simulink model "cop"  (R2020a)
settings: Solver=FixedStepAuto  StartTime=0.0  StopTime=300  FixedStep=1  RelTol=1e-3
undefined symbols (not defined in the file or in its folder): inf_depth, Kc_ini, PGravel
libraries: simulink x4
(part 2 of 2)

== system cop/COP/Climate Model/ Final Calculation for Data/Wind Speed/Wind Speed measured at 2m height (u2) [m//s] ==
  uz : Inport
  z : Inport  Port=2
  Constant : Constant  Value=4.87
  Constant1 : Constant  Value=67.8
  Constant2 : Constant  Value=5.42
  Divide : Product  Inputs=**/
  Math Function : Math  Operator=log  SaturateOnIntegerOverflow=on
  Product : Product
  Subtract : Sum  Inputs=+-
  u2 : Outport
  wires:
  uz/1 -> Divide/1
  Constant/1 -> Divide/2
  Math Function/1 -> Divide/3
  z/1 -> Product/2
  Constant1/1 -> Product/1
  Product/1 -> Subtract/1
  Subtract/1 -> Math Function/1
  Constant2/1 -> Subtract/2
  Divide/1 -> u2/1

== system cop/COP/Soil Model/Dual Crop Coefficient (Kcb + Ke)/Crop Basal Component/Adjustment to Crop Coefficient ==
  Constant2 : Constant  Value=0.3
  Constant3 : Constant  Value=3
  Constant4 : Constant  Value=0.004
  Constant5 : Constant  Value=45
  Constant6 : Constant  Value=0.04
  Constant7 : Constant  Value=2
  Divide : Product  Inputs=*/
  Math Function : Math  Operator=pow  SaturateOnIntegerOverflow=on
  Product : Product
  Product1 : Product
  Product2 : Product
  Subtract : Sum  Inputs=+-
  Subtract1 : Sum  Inputs=+-
  Subtract2 : Sum  Inputs=+-
  Kcb_adj : Outport
  wires:
  Product/1 -> Kcb_adj/1
  Subtract/1 -> Product/1
  [u2] -> Subtract2/1
  Constant4/1 -> Product1/1
  Constant7/1 -> Subtract2/2
  [RHmin] -> Subtract1/1
  Product1/1 -> Subtract/2
  Constant5/1 -> Subtract1/2
  Divide/1 -> Math Function/1
  Constant3/1 -> Divide/2
  Constant2/1 -> Math Function/2
  Product2/1 -> Subtract/1
  [MaxCropHatStage] -> Divide/1
  Subtract2/1 -> Product2/2
  Math Function/1 -> Product/2
  Subtract1/1 -> Product1/2
  Constant6/1 -> Product2/1

== system cop/COP/Soil Model/Dual Crop Coefficient (Kcb + Ke)/Crop Basal Component/Development Stage ==
  Kcb ini : Inport
  Kcb mid : Inport  Port=2
  Add : Sum
  Divide : Product  Inputs=*/
  Product : Product
  Subtract : Sum  Inputs=+-
  Subtract1 : Sum  Inputs=+-
  Out1 : Outport
  wires:
  Add/1 -> Out1/1
  Kcb ini/1 -> Add/1, Subtract/2
  Product/1 -> Add/2
  Subtract/1 -> Product/2
  Kcb mid/1 -> Subtract/1
  Divide/1 -> Product/1
  [Ldev] -> Divide/2
  Subtract1/1 -> Divide/1
  [Lini] -> Subtract1/2
  [DafterPD] -> Subtract1/1

== system cop/COP/Soil Model/Dual Crop Coefficient (Kcb + Ke)/Crop Basal Component/Late Season Stage ==
  Kcb mid : Inport
  Kcb_adj : Inport  Port=2
  Add : Sum
  Add1 : Sum
  Add2 : Sum  Inputs=+++
  Divide : Product  Inputs=*/
  Product : Product
  Subtract : Sum  Inputs=+-
  Subtract1 : Sum  Inputs=+-
  Out1 : Outport
  wires:
  [Kcb_end] -> Add/1
  Kcb_adj/1 -> Add/2
  Subtract/1 -> Product/2
  Divide/1 -> Product/1
  [DafterPD] -> Subtract1/1
  Add1/1 -> Out1/1
  Product/1 -> Add1/2
  [Llate] -> Divide/2
  Kcb mid/1 -> Add1/1, Subtract/2
  Subtract1/1 -> Divide/1
  Add/1 -> Subtract/1
  Add2/1 -> Subtract1/2
  [Lini] -> Add2/1
  [Ldev] -> Add2/2
  [Lmid] -> Add2/3

== system cop/COP/Soil Model/Dual Crop Coefficient (Kcb + Ke)/Crop Basal Component/Mid-season Stage ==
  Kcb_adj : Inport
  Add : Sum
  Constant : Constant  Value=0
  Switch : Switch  Criteria=u2 > Threshold  Threshold=0.45
  Kcb mid : Outport
  wires:
  Add/1 -> Kcb mid/1
  [Kcb_mid] -> Add/1, Switch/2
  Kcb_adj/1 -> Switch/1
  Switch/1 -> Add/2
  Constant/1 -> Switch/3

== system cop/COP/Soil Model/Dual Crop Coefficient (Kcb + Ke)/Evaporation Component/Exposed and wetted soil fraction (few) ==
  Constant1 : Constant
  Effective fraction of soil surface covered by vegetation fc : Subsystem
  Min : MinMax  Inputs=2
  Subtract : Sum  Inputs=+-
  Out1 : Outport
  wires:
  Min/1 -> Out1/1
  Subtract/1 -> Min/1
  [fw] -> Min/2
  Constant1/1 -> Subtract/1
  Effective fraction of soil surface covered by vegetation fc/1(Out1) -> Subtract/2

== system cop/COP/Soil Model/Dual Crop Coefficient (Kcb + Ke)/Evaporation Component/Soil evaporation reduction coefficient (Kr) ==
  De_i Daily Water Balance [mm] : Subsystem
  Delay : Delay  DelayLength=1  InitialConditionSource=Input port  InitialCondition=0
      settings: InputPortMap=u0,p4
  Display : Display
  Divide : Product  Inputs=*/
  REWmax total readily evaporable water [mm] : Subsystem
  Subtract : Sum  Inputs=+-
  Subtract1 : Sum  Inputs=+-
  TEWmax total evaporable water [mm] : Subsystem
  initial De_i-1 value : Constant  Value=0
  Out1 : Outport
  tag scope: De_past=global, REW=global, TEW=global
  wires:
  Divide/1 -> Out1/1
  TEWmax total evaporable water [mm]/1(Out1) -> Display/1, [TEW], Subtract/1, Subtract1/1
  Subtract/1 -> Divide/1
  Subtract1/1 -> Divide/2
  REWmax total readily evaporable water [mm]/1(Out1) -> [REW], Subtract1/2
  [De_past] -> Subtract/2
  De_i Daily Water Balance [mm]/1(Out1) -> Delay/1
  Delay/1 -> De_i Daily Water Balance [mm]/1(De_past), [De_past]
  initial De_i-1 value/1 -> Delay/2

== system cop/COP/Soil Model/Dual Crop Coefficient (Kcb + Ke)/Evaporation Component/Upper Limit (Kc max) ==
  Kcb : Inport
  0.05 : Constant  Value=0.05
  Add : Sum
  Add1 : Sum
  Adjustment to Crop Coefficient : Subsystem
  Constant : Constant  Value=1.2
  MinMax : MinMax  Function=max  Inputs=2
  Out1 : Outport
  wires:
  MinMax/1 -> Out1/1
  Constant/1 -> Add/1
  Adjustment to Crop Coefficient/1(Kcb_adj) -> Add/2
  Add/1 -> MinMax/1
  Kcb/1 -> Add1/1
  Add1/1 -> MinMax/2
  0.05/1 -> Add1/2

== system cop/COP/Soil Model/Reference Evapotraspiration (ET0) [mm//day]/Actual Vapor Pressure (ea) [kPa]/Derived from Dewpoint Temperature ==
  Saturation Vapor Pressure (eo) : Subsystem
  Out1 : Outport
  wires:
  [Tdew] -> Saturation Vapor Pressure (eo)/1(In1)
  Saturation Vapor Pressure (eo)/1(Out1) -> Out1/1

== system cop/COP/Soil Model/Reference Evapotraspiration (ET0) [mm//day]/Actual Vapor Pressure (ea) [kPa]/Derived from Psychrometric Data ==
  Constant : Constant  Value=apsy
  Product : Product
  Product1 : Product
  Saturation Vapor Pressure (eo) : Subsystem
  Subtract : Sum  Inputs=+-
  Subtract1 : Sum  Inputs=+-
  Out1 : Outport
  wires:
  Subtract/1 -> Out1/1
  Saturation Vapor Pressure (eo)/1(Out1) -> Subtract/1
  [Twet] -> Subtract1/2, Saturation Vapor Pressure (eo)/1(In1)
  [Tdry] -> Subtract1/1
  Subtract1/1 -> Product/1
  Product/1 -> Subtract/2
  Product1/1 -> Product/2
  [AP] -> Product1/2
  Constant/1 -> Product1/1

== system cop/COP/Soil Model/Reference Evapotraspiration (ET0) [mm//day]/Actual Vapor Pressure (ea) [kPa]/Derived from RHmax & RHmin ==
  Add : Sum
  Constant : Constant  Value=100
  Constant1 : Constant  Value=2
  Constant2 : Constant  Value=100
  Divide : Product  Inputs=**/
  Divide1 : Product  Inputs=**/
  Divide2 : Product  Inputs=*/
  Saturation Vapor Pressure (eo) : Subsystem
  Saturation Vapor Pressure (eo)1 : Subsystem
  Out1 : Outport
  wires:
  Divide2/1 -> Out1/1
  [Tmin] -> Saturation Vapor Pressure (eo)/1(In1)
  Saturation Vapor Pressure (eo)/1(Out1) -> Divide/1
  [RHmax] -> Divide/2
  Constant/1 -> Divide/3
  Divide/1 -> Add/1
  Divide1/1 -> Add/2
  Add/1 -> Divide2/1
  Constant1/1 -> Divide2/2
  Constant2/1 -> Divide1/3
  [RHmin] -> Divide1/2
  [Tmax] -> Saturation Vapor Pressure (eo)1/1(In1)
  Saturation Vapor Pressure (eo)1/1(Out1) -> Divide1/1

== system cop/COP/Soil Model/Reference Evapotraspiration (ET0) [mm//day]/Actual Vapor Pressure (ea) [kPa]/Derived from RHmax only ==
  Constant : Constant  Value=100
  Divide : Product  Inputs=**/
  Saturation Vapor Pressure (eo) : Subsystem
  Out1 : Outport
  wires:
  Constant/1 -> Divide/3
  [Tmin] -> Saturation Vapor Pressure (eo)/1(In1)
  [RHmax] -> Divide/2
  Saturation Vapor Pressure (eo)/1(Out1) -> Divide/1
  Divide/1 -> Out1/1

== system cop/COP/Soil Model/Reference Evapotraspiration (ET0) [mm//day]/Actual Vapor Pressure (ea) [kPa]/Derived from RHmean only ==
  Add : Sum
  Constant : Constant  Value=2
  Constant1 : Constant  Value=100
  Divide : Product  Inputs=*/
  Divide1 : Product  Inputs=*/
  Product : Product
  Saturation Vapor Pressure (eo) : Subsystem
  Saturation Vapor Pressure (eo)1 : Subsystem
  Out1 : Outport
  wires:
  [Tmax] -> Saturation Vapor Pressure (eo)/1(In1)
  Saturation Vapor Pressure (eo)/1(Out1) -> Add/1
  Saturation Vapor Pressure (eo)1/1(Out1) -> Add/2
  [Tmin] -> Saturation Vapor Pressure (eo)1/1(In1)
  Add/1 -> Divide/1
  Constant/1 -> Divide/2
  Divide/1 -> Product/2
  [RHmean] -> Divide1/1
  Constant1/1 -> Divide1/2
  Divide1/1 -> Product/1
  Product/1 -> Out1/1

== system cop/COP/Soil Model/Reference Evapotraspiration (ET0) [mm//day]/Mean Saturation Vapor Pressure (es) [kPa] /Saturation Vapor Pressure (eo) ==
  In1 : Inport
  Add : Sum
  Constant : Constant  Value=0.6108
  Constant1 : Constant  Value=17.27
  Constant2 : Constant  Value=237.3
  Divide : Product  Inputs=**/
  Math Function : Math  SaturateOnIntegerOverflow=on
  Product : Product
  Out1 : Outport
  wires:
  Product/1 -> Out1/1
  Constant1/1 -> Divide/1
  In1/1 -> Add/1, Divide/2
  Add/1 -> Divide/3
  Divide/1 -> Math Function/1
  Constant/1 -> Product/1
  Constant2/1 -> Add/2
  Math Function/1 -> Product/2

== system cop/COP/Soil Model/Reference Evapotraspiration (ET0) [mm//day]/Mean Saturation Vapor Pressure (es) [kPa] /Saturation Vapor Pressure (eo) 2 ==
  In1 : Inport
  Add1 : Sum
  Constant3 : Constant  Value=0.6108
  Constant4 : Constant  Value=17.27
  Constant5 : Constant  Value=237.3
  Divide1 : Product  Inputs=**/
  Math Function1 : Math  SaturateOnIntegerOverflow=on
  Product1 : Product
  Out1 : Outport
  wires:
  Math Function1/1 -> Product1/2
  Constant4/1 -> Divide1/1
  Add1/1 -> Divide1/3
  Constant3/1 -> Product1/1
  Divide1/1 -> Math Function1/1
  In1/1 -> Divide1/2, Add1/1
  Product1/1 -> Out1/1
  Constant5/1 -> Add1/2

== system cop/COP/Soil Model/Reference Evapotraspiration (ET0) [mm//day]/Psychrometric Constant (Y) [kPA//°C]/Latent Heat of Vaporization (l) [MJ//kg] ==
  "Latent Heat for an Air Temperature of about 20°C " : Constant  Value=2.45
  l : Outport
  wires:
  "Latent Heat for an Air Temperature of about 20°C "/1 -> l/1

== system cop/COP/Soil Model/Reference Evapotraspiration (ET0) [mm//day]/Soil Heat Flux Density (G) [MJ//m^2//day]/Long Time Steps ==
  Divide : Product  Inputs=**/*
  Subtract : Sum  Inputs=+-
  Out1 : Outport
  wires:
  [cs] -> Divide/1
  [Tmean] -> Subtract/1
  [Tpast] -> Subtract/2
  Subtract/1 -> Divide/2
  [Tpast_t] -> Divide/3
  [Zr] -> Divide/4
  Divide/1 -> Out1/1

== system cop/COP/Soil Model/Soil Data Calculation/Estimated Soil Heat Capacity (UC Davis)/Bulk Density (Saxton and Rawls Function) [g//cm^3) ==
  Add : Sum
  Constant : Constant
  Constant1 : Constant  Value=2.65
  Normal Density (g/cm^3) : Subsystem
  Product : Product
  Product1 : Product
  Subtract : Sum  Inputs=+-
  Volum Fraction of Gravel (g/cm^3) : Subsystem
  Out1 : Outport
  wires:
  Add/1 -> Out1/1
  Normal Density (g/cm^3)/1(Out1) -> Product/1, Volum Fraction of Gravel (g/cm^3)/1(In1)
  Subtract/1 -> Product/2
  Product/1 -> Add/1
  Constant/1 -> Subtract/1
  Product1/1 -> Add/2
  Constant1/1 -> Product1/2
  Volum Fraction of Gravel (g/cm^3)/1(Out1) -> Subtract/2, Product1/1

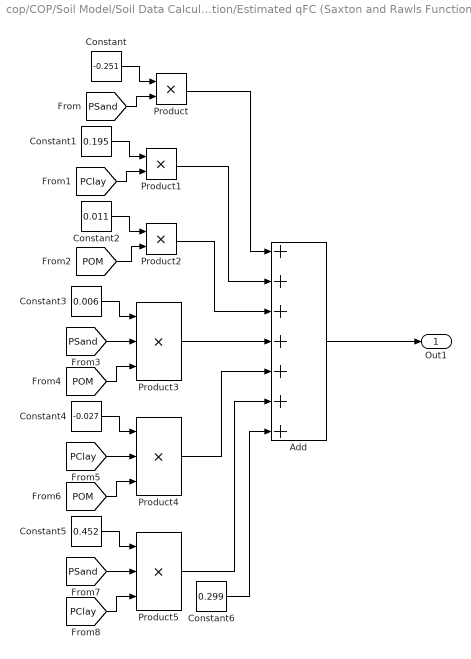
== system cop/COP/Soil Model/Soil Data Calculation/Estimated qFC (Saxton and Rawls Function)/θ33t ==
  Add : Sum  Inputs=+++++++
  Constant : Constant  Value=-0.251
  Constant1 : Constant  Value=0.195
  Constant2 : Constant  Value=0.011
  Constant3 : Constant  Value=0.006
  Constant4 : Constant  Value=-0.027
  Constant5 : Constant  Value=0.452
  Constant6 : Constant  Value=0.299
  Product : Product
  Product1 : Product
  Product2 : Product
  Product3 : Product  Inputs=3
  Product4 : Product  Inputs=3
  Product5 : Product  Inputs=3
  Out1 : Outport
  wires:
  [PClay] -> Product5/3
  [PClay] -> Product1/2
  Constant4/1 -> Product4/1
  Product1/1 -> Add/2
  Constant3/1 -> Product3/1
  Product5/1 -> Add/6
  [PClay] -> Product4/2
  Product4/1 -> Add/5
  Constant6/1 -> Add/7
  Constant5/1 -> Product5/1
  [PSand] -> Product5/2
  Product/1 -> Add/1
  [PSand] -> Product/2
  Product2/1 -> Add/3
  Constant2/1 -> Product2/1
  Constant1/1 -> Product1/1
  Product3/1 -> Add/4
  Constant/1 -> Product/1
  [POM] -> Product2/2
  [PSand] -> Product3/2
  [POM] -> Product4/3
  [POM] -> Product3/3
  Add/1 -> Out1/1

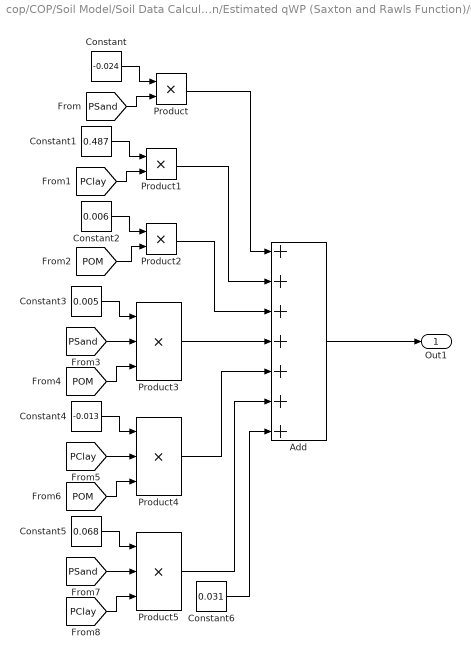
== system cop/COP/Soil Model/Soil Data Calculation/Estimated qWP (Saxton and Rawls Function)/θ1500t ==
  Add : Sum  Inputs=+++++++
  Constant : Constant  Value=-0.024
  Constant1 : Constant  Value=0.487
  Constant2 : Constant  Value=0.006
  Constant3 : Constant  Value=0.005
  Constant4 : Constant  Value=-0.013
  Constant5 : Constant  Value=0.068
  Constant6 : Constant  Value=0.031
  Product : Product
  Product1 : Product
  Product2 : Product
  Product3 : Product  Inputs=3
  Product4 : Product  Inputs=3
  Product5 : Product  Inputs=3
  Out1 : Outport
  wires:
  [PClay] -> Product5/3
  [PClay] -> Product1/2
  Constant4/1 -> Product4/1
  Product1/1 -> Add/2
  Constant3/1 -> Product3/1
  Product5/1 -> Add/6
  [PClay] -> Product4/2
  Product4/1 -> Add/5
  Constant6/1 -> Add/7
  Constant5/1 -> Product5/1
  [PSand] -> Product5/2
  Product/1 -> Add/1
  [PSand] -> Product/2
  Product2/1 -> Add/3
  Constant2/1 -> Product2/1
  Constant1/1 -> Product1/1
  Product3/1 -> Add/4
  Constant/1 -> Product/1
  [POM] -> Product2/2
  [PSand] -> Product3/2
  [POM] -> Product4/3
  [POM] -> Product3/3
  Add/1 -> Out1/1

== system cop/COP/Climate Model/ Final Calculation for Data/Net Radiation at the Crop Surface (Rn) [MJ//m^2//day]/Extraterrestrial Radiation (Ra) [MJ//m^2//day]/Inverse Relative Distance Earth-Sun (dr) ==
  J : Inport
  Add : Sum
  Constant : Constant
  Constant1 : Constant  Value=0.033
  Constant2 : Constant  Value=2*pi
  Divide : Product  Inputs=**/
  Product : Product
  Trigonometric Function : Trigonometry  Operator=cos
  dr : Outport
  wires:
  Add/1 -> dr/1
  Constant/1 -> Add/1
  Product/1 -> Add/2
  Constant1/1 -> Product/1
  Trigonometric Function/1 -> Product/2
  Divide/1 -> Trigonometric Function/1
  Constant2/1 -> Divide/1
  [DinYear] -> Divide/3
  J/1 -> Divide/2

== system cop/COP/Climate Model/ Final Calculation for Data/Net Radiation at the Crop Surface (Rn) [MJ//m^2//day]/Extraterrestrial Radiation (Ra) [MJ//m^2//day]/Latitude in Radian (φ) [rad] ==
  Add : Sum
  Constant : Constant  Value=pi/180
  Constant1 : Constant  Value=60
  Divide : Product  Inputs=*/
  Product : Product
  φ : Outport
  wires:
  Constant/1 -> Product/1
  Add/1 -> Product/2
  [LatDeg] -> Add/1
  [LatMin] -> Divide/1
  Constant1/1 -> Divide/2
  Divide/1 -> Add/2
  Product/1 -> φ/1

== system cop/COP/Climate Model/ Final Calculation for Data/Net Radiation at the Crop Surface (Rn) [MJ//m^2//day]/Extraterrestrial Radiation (Ra) [MJ//m^2//day]/Solar Declination in Radian (δ) [rad] ==
  J : Inport
  Constant1 : Constant  Value=0.409
  Constant2 : Constant  Value=2*pi
  Constant4 : Constant  Value=1.39
  Divide : Product  Inputs=**/
  Product : Product
  Subtract : Sum  Inputs=+-
  Trigonometric Function : Trigonometry
  δ : Outport
  wires:
  [DinYear] -> Divide/3
  Product/1 -> δ/1
  Trigonometric Function/1 -> Product/2
  J/1 -> Divide/2
  Constant2/1 -> Divide/1
  Constant1/1 -> Product/1
  Divide/1 -> Subtract/1
  Subtract/1 -> Trigonometric Function/1
  Constant4/1 -> Subtract/2

== system cop/COP/Climate Model/ Final Calculation for Data/Net Radiation at the Crop Surface (Rn) [MJ//m^2//day]/Extraterrestrial Radiation (Ra) [MJ//m^2//day]/Sunset Hour Angle (Ws) [rad] ==
  Constant : Constant  Value=-1
  Product : Product  Inputs=3
  Trigonometric Function : Trigonometry  Operator=acos
  Trigonometric Function1 : Trigonometry  Operator=tan
  Trigonometric Function2 : Trigonometry  Operator=tan
  Ws : Outport
  wires:
  Trigonometric Function/1 -> Ws/1
  Product/1 -> Trigonometric Function/1
  Constant/1 -> Product/1
  Trigonometric Function1/1 -> Product/2
  Trigonometric Function2/1 -> Product/3
  [LatRad] -> Trigonometric Function1/1
  [SolDec] -> Trigonometric Function2/1

== system cop/COP/Climate Model/ Final Calculation for Data/Net Radiation at the Crop Surface (Rn) [MJ//m^2//day]/Net Solar//Shortwave Radiation (Rns) [MJ//m^2//day]/Albedo or canopy reflection coefficient for the reference crop (G) ==
  Constant : Constant  Value=0.23
  Out1 : Outport
  wires:
  Constant/1 -> Out1/1

== system cop/COP/Climate Model/ Final Calculation for Data/Net Radiation at the Crop Surface (Rn) [MJ//m^2//day]/Solar Radiation (Rs) [MJ//m^2//day]/Angstrom Formula if AI_Rs not avaliable ==
  In1 : Inport
  Add : Sum
  Default as : Constant  Value=0.25
  Default bs : Constant  Value=0.50
  Divide : Product  Inputs=**/
  Maximum Daylight Hour (N) [hour] : Subsystem
  Product : Product
  Out1 : Outport
  wires:
  Default as/1 -> Add/1
  Default bs/1 -> Divide/1
  Divide/1 -> Add/2
  In1/1 -> Divide/2
  Add/1 -> Product/1
  Product/1 -> Out1/1
  [Ra] -> Product/2
  Maximum Daylight Hour (N) [hour]/1(N) -> Divide/3

== system cop/COP/Climate Model/ Final Calculation for Data/Net Radiation at the Crop Surface (Rn) [MJ//m^2//day]/Solar Radiation (Rs) [MJ//m^2//day]/Hargreaves Formula if AI_Rs and hour of daylight is not available ==
  Constant : Constant  Value=kRs
  Product : Product  Inputs=3
  Sqrt : Sqrt  SaturateOnIntegerOverflow=on
  Subtract : Sum  Inputs=+-
  Rs : Outport
  wires:
  Product/1 -> Rs/1
  Constant/1 -> Product/1
  [Ra] -> Product/3
  Sqrt/1 -> Product/2
  Subtract/1 -> Sqrt/1
  [Tmin] -> Subtract/2
  [Tmax] -> Subtract/1

== system cop/COP/Soil Model/Dual Crop Coefficient (Kcb + Ke)/Evaporation Component/Exposed and wetted soil fraction (few)/Effective fraction of soil surface covered by vegetation fc ==
  Constant : Constant
  Constant1 : Constant  Value=0.5
  Constant2 : Constant  Value=0.01
  Divide : Product  Inputs=*/
  Math Function : Math  Operator=pow  SaturateOnIntegerOverflow=on
  MinMax : MinMax  Function=max  Inputs=2
  Product : Product
  Subtract : Sum  Inputs=+-
  Subtract1 : Sum  Inputs=+-
  Subtract2 : Sum
  Out1 : Outport
  wires:
  Divide/1 -> Math Function/1
  [Kcb] -> Subtract/1
  [Kcb_ini] -> Subtract1/2, Subtract/2
  Subtract/1 -> MinMax/2
  [Kc_max] -> Subtract1/1
  Subtract1/1 -> Divide/2
  Subtract2/1 -> Math Function/2
  Constant/1 -> Subtract2/1
  Product/1 -> Subtract2/2
  Constant1/1 -> Product/1
  [Ph] -> Product/2
  Math Function/1 -> Out1/1
  MinMax/1 -> Divide/1
  Constant2/1 -> MinMax/1

== system cop/COP/Soil Model/Dual Crop Coefficient (Kcb + Ke)/Evaporation Component/Soil evaporation reduction coefficient (Kr)/De_i Daily Water Balance [mm] ==
  De_past : Inport
  Constant : Constant  Value=0
  Constant1 : Constant  Value=0
  Deep Percolation DPe [mm/day] : Subsystem
  Divide : Product  Inputs=*/
  Divide1 : Product  Inputs=*/
  MinMax : MinMax  Inputs=2
  MinMax1 : MinMax  Function=max  Inputs=2
  MinMax2 : MinMax  Function=max  Inputs=2
  Subtract : Sum  Inputs=+--+++
  Subtract1 : Sum  Inputs=+-
  Out1 : Outport
  wires:
  De_past/1 -> Subtract/1
  Subtract/1 -> MinMax/1
  [P] -> Subtract1/1
  [RO] -> Subtract1/2
  Subtract1/1 -> Subtract/2
  [I] -> Divide/1
  Divide/1 -> Subtract/3
  [fw] -> Divide/2
  Divide1/1 -> Subtract/4
  [E] -> Divide1/1
  [few] -> Divide1/2
  [Te] -> Subtract/5
  Deep Percolation DPe [mm/day]/1(Out1) -> MinMax2/1
  MinMax/1 -> MinMax1/1
  MinMax1/1 -> Out1/1
  [TEW] -> MinMax/2
  Constant/1 -> MinMax1/2
  Constant1/1 -> MinMax2/2
  MinMax2/1 -> Subtract/6

== system cop/COP/Soil Model/Dual Crop Coefficient (Kcb + Ke)/Evaporation Component/Soil evaporation reduction coefficient (Kr)/REWmax total readily evaporable water [mm] ==
  MABIA Method : Subsystem
  Manual Switch : ManualSwitch  CurrentSetting=0
  Ritchie et al. (1989) : Subsystem
  Out1 : Outport
  wires:
  MABIA Method/1(Out1) -> Manual Switch/2
  Ritchie et al. (1989)/1(Out1) -> Manual Switch/1
  Manual Switch/1 -> Out1/1

== system cop/COP/Soil Model/Dual Crop Coefficient (Kcb + Ke)/Evaporation Component/Soil evaporation reduction coefficient (Kr)/TEWmax total evaporable water [mm] ==
  Constant : Constant  Value=1000
  Constant1 : Constant  Value=0.5
  Product : Product  Inputs=3
  Product1 : Product
  Subtract : Sum  Inputs=+-
  Out1 : Outport
  wires:
  Product/1 -> Out1/1
  Constant/1 -> Product/1
  Subtract/1 -> Product/2
  [qFC] -> Subtract/1
  Product1/1 -> Subtract/2
  [qWP] -> Product1/2
  Constant1/1 -> Product1/1
  [Ze] -> Product/3

== system cop/COP/Soil Model/Dual Crop Coefficient (Kcb + Ke)/Evaporation Component/Upper Limit (Kc max)/Adjustment to Crop Coefficient ==
  Constant2 : Constant  Value=0.3
  Constant3 : Constant  Value=3
  Constant4 : Constant  Value=0.004
  Constant5 : Constant  Value=45
  Constant6 : Constant  Value=0.04
  Constant7 : Constant  Value=2
  Divide : Product  Inputs=*/
  Math Function : Math  Operator=pow  SaturateOnIntegerOverflow=on
  Product : Product
  Product1 : Product
  Product2 : Product
  Subtract : Sum  Inputs=+-
  Subtract1 : Sum  Inputs=+-
  Subtract2 : Sum  Inputs=+-
  Kcb_adj : Outport
  wires:
  Product/1 -> Kcb_adj/1
  Subtract/1 -> Product/1
  [u2] -> Subtract2/1
  Constant4/1 -> Product1/1
  Constant7/1 -> Subtract2/2
  [RHmin] -> Subtract1/1
  Product1/1 -> Subtract/2
  Constant5/1 -> Subtract1/2
  Divide/1 -> Math Function/1
  Constant3/1 -> Divide/2
  Constant2/1 -> Math Function/2
  Product2/1 -> Subtract/1
  [MaxCropHatStage] -> Divide/1
  Subtract2/1 -> Product2/2
  Math Function/1 -> Product/2
  Subtract1/1 -> Product1/2
  Constant6/1 -> Product2/1

== system cop/COP/Soil Model/Reference Evapotraspiration (ET0) [mm//day]/Actual Vapor Pressure (ea) [kPa]/Derived from Dewpoint Temperature/Saturation Vapor Pressure (eo) ==
  In1 : Inport
  Add : Sum
  Constant : Constant  Value=0.6108
  Constant1 : Constant  Value=17.27
  Constant2 : Constant  Value=237.3
  Divide : Product  Inputs=**/
  Math Function : Math  SaturateOnIntegerOverflow=on
  Product : Product
  Out1 : Outport
  wires:
  Product/1 -> Out1/1
  Constant1/1 -> Divide/1
  In1/1 -> Add/1, Divide/2
  Add/1 -> Divide/3
  Divide/1 -> Math Function/1
  Constant/1 -> Product/1
  Constant2/1 -> Add/2
  Math Function/1 -> Product/2

== system cop/COP/Soil Model/Reference Evapotraspiration (ET0) [mm//day]/Actual Vapor Pressure (ea) [kPa]/Derived from Psychrometric Data/Saturation Vapor Pressure (eo) ==
  In1 : Inport
  Add : Sum
  Constant : Constant  Value=0.6108
  Constant1 : Constant  Value=17.27
  Constant2 : Constant  Value=237.3
  Divide : Product  Inputs=**/
  Math Function : Math  SaturateOnIntegerOverflow=on
  Product : Product
  Out1 : Outport
  wires:
  Product/1 -> Out1/1
  Constant1/1 -> Divide/1
  In1/1 -> Add/1, Divide/2
  Add/1 -> Divide/3
  Divide/1 -> Math Function/1
  Constant/1 -> Product/1
  Constant2/1 -> Add/2
  Math Function/1 -> Product/2

== system cop/COP/Soil Model/Reference Evapotraspiration (ET0) [mm//day]/Actual Vapor Pressure (ea) [kPa]/Derived from RHmax & RHmin/Saturation Vapor Pressure (eo) ==
  In1 : Inport
  Add : Sum
  Constant : Constant  Value=0.6108
  Constant1 : Constant  Value=17.27
  Constant2 : Constant  Value=237.3
  Divide : Product  Inputs=**/
  Math Function : Math  SaturateOnIntegerOverflow=on
  Product : Product
  Out1 : Outport
  wires:
  Product/1 -> Out1/1
  Constant1/1 -> Divide/1
  In1/1 -> Add/1, Divide/2
  Add/1 -> Divide/3
  Divide/1 -> Math Function/1
  Constant/1 -> Product/1
  Constant2/1 -> Add/2
  Math Function/1 -> Product/2

== system cop/COP/Soil Model/Reference Evapotraspiration (ET0) [mm//day]/Actual Vapor Pressure (ea) [kPa]/Derived from RHmax & RHmin/Saturation Vapor Pressure (eo)1 ==
  In1 : Inport
  Add : Sum
  Constant : Constant  Value=0.6108
  Constant1 : Constant  Value=17.27
  Constant2 : Constant  Value=237.3
  Divide : Product  Inputs=**/
  Math Function : Math  SaturateOnIntegerOverflow=on
  Product : Product
  Out1 : Outport
  wires:
  Math Function/1 -> Product/2
  Constant2/1 -> Add/2
  Constant/1 -> Product/1
  Divide/1 -> Math Function/1
  Add/1 -> Divide/3
  In1/1 -> Divide/2, Add/1
  Constant1/1 -> Divide/1
  Product/1 -> Out1/1

== system cop/COP/Soil Model/Reference Evapotraspiration (ET0) [mm//day]/Actual Vapor Pressure (ea) [kPa]/Derived from RHmax only/Saturation Vapor Pressure (eo) ==
  In1 : Inport
  Add : Sum
  Constant : Constant  Value=0.6108
  Constant1 : Constant  Value=17.27
  Constant2 : Constant  Value=237.3
  Divide : Product  Inputs=**/
  Math Function : Math  SaturateOnIntegerOverflow=on
  Product : Product
  Out1 : Outport
  wires:
  Product/1 -> Out1/1
  Constant1/1 -> Divide/1
  In1/1 -> Add/1, Divide/2
  Add/1 -> Divide/3
  Divide/1 -> Math Function/1
  Constant/1 -> Product/1
  Constant2/1 -> Add/2
  Math Function/1 -> Product/2

== system cop/COP/Soil Model/Reference Evapotraspiration (ET0) [mm//day]/Actual Vapor Pressure (ea) [kPa]/Derived from RHmean only/Saturation Vapor Pressure (eo) ==
  In1 : Inport
  Add : Sum
  Constant : Constant  Value=0.6108
  Constant1 : Constant  Value=17.27
  Constant2 : Constant  Value=237.3
  Divide : Product  Inputs=**/
  Math Function : Math  SaturateOnIntegerOverflow=on
  Product : Product
  Out1 : Outport
  wires:
  Product/1 -> Out1/1
  Constant1/1 -> Divide/1
  In1/1 -> Add/1, Divide/2
  Add/1 -> Divide/3
  Divide/1 -> Math Function/1
  Constant/1 -> Product/1
  Constant2/1 -> Add/2
  Math Function/1 -> Product/2

== system cop/COP/Soil Model/Reference Evapotraspiration (ET0) [mm//day]/Actual Vapor Pressure (ea) [kPa]/Derived from RHmean only/Saturation Vapor Pressure (eo)1 ==
  In1 : Inport
  Add : Sum
  Constant : Constant  Value=0.6108
  Constant1 : Constant  Value=17.27
  Constant2 : Constant  Value=237.3
  Divide : Product  Inputs=**/
  Math Function : Math  SaturateOnIntegerOverflow=on
  Product : Product
  Out1 : Outport
  wires:
  Math Function/1 -> Product/2
  Constant2/1 -> Add/2
  Constant/1 -> Product/1
  Divide/1 -> Math Function/1
  Add/1 -> Divide/3
  In1/1 -> Divide/2, Add/1
  Constant1/1 -> Divide/1
  Product/1 -> Out1/1

== system cop/COP/Soil Model/Soil Data Calculation/Estimated Soil Heat Capacity (UC Davis)/Bulk Density (Saxton and Rawls Function) [g//cm^3)/Normal Density (g//cm^3) ==
  Constant : Constant  Value=2.65
  Constant1 : Constant
  Product : Product
  Saturated Moisture θS : Subsystem
  Subtract : Sum  Inputs=+-
  Out1 : Outport
  wires:
  Product/1 -> Out1/1
  Constant/1 -> Product/2
  Subtract/1 -> Product/1
  Constant1/1 -> Subtract/1
  Saturated Moisture θS/1(Out1) -> Subtract/2

== system cop/COP/Soil Model/Soil Data Calculation/Estimated Soil Heat Capacity (UC Davis)/Bulk Density (Saxton and Rawls Function) [g//cm^3)/Volum Fraction of Gravel (g//cm^3) ==
  In1 : Inport
  Constant : Constant  Value=2.65
  Constant1 : Constant
  Constant2 : Constant
  Divide : Product  Inputs=*/
  Divide1 : Product  Inputs=*/
  Product : Product
  Product1 : Product
  Subtract : Sum  Inputs=+-
  Subtract1 : Sum  Inputs=+-
  Out1 : Outport
  wires:
  In1/1 -> Divide/1
  [PGravel] -> Product1/1, Product/2
  Constant/1 -> Divide/2
  Divide/1 -> Subtract1/2, Product/1
  Product/1 -> Divide1/1
  Subtract/1 -> Divide1/2
  Constant1/1 -> Subtract/1
  Product1/1 -> Subtract/2
  Subtract1/1 -> Product1/2
  Constant2/1 -> Subtract1/1
  Divide1/1 -> Out1/1

== system cop/COP/Climate Model/ Final Calculation for Data/Net Radiation at the Crop Surface (Rn) [MJ//m^2//day]/Solar Radiation (Rs) [MJ//m^2//day]/Angstrom Formula if AI_Rs not avaliable/Maximum Daylight Hour (N) [hour] ==
  Constant : Constant  Value=24
  Constant1 : Constant  Value=pi
  Divide : Product  Inputs=**/
  N : Outport
  wires:
  Divide/1 -> N/1
  [Ws] -> Divide/2
  Constant/1 -> Divide/1
  Constant1/1 -> Divide/3

== system cop/COP/Soil Model/Dual Crop Coefficient (Kcb + Ke)/Evaporation Component/Soil evaporation reduction coefficient (Kr)/De_i Daily Water Balance [mm]/Deep Percolation DPe [mm//day] ==
  Add : Sum  Inputs=++-
  Divide : Product  Inputs=*/
  Subtract : Sum  Inputs=+-
  Out1 : Outport
  wires:
  Divide/1 -> Add/2
  [P] -> Subtract/1
  [RO] -> Subtract/2
  Subtract/1 -> Add/1
  [I] -> Divide/1
  [fw] -> Divide/2
  [De_past] -> Add/3
  Add/1 -> Out1/1

== system cop/COP/Soil Model/Dual Crop Coefficient (Kcb + Ke)/Evaporation Component/Soil evaporation reduction coefficient (Kr)/REWmax total readily evaporable water [mm]/MABIA Method ==
  Add : Sum
  Constant : Constant  Value=3.121
  Constant1 : Constant  Value=22.896
  Product : Product
  Product1 : Product
  Out1 : Outport
  wires:
  Product1/1 -> Out1/1
  Constant/1 -> Product/1
  [TEW] -> Product/2
  Product/1 -> Add/1
  Constant1/1 -> Add/2
  Add/1 -> Product1/1
  [Ze] -> Product1/2

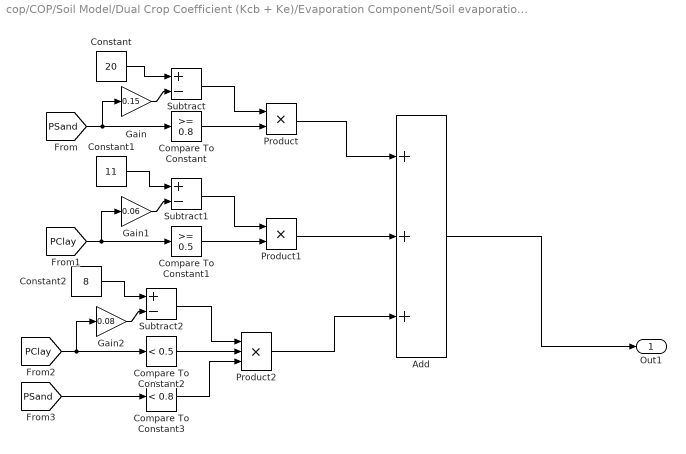
== system cop/COP/Soil Model/Dual Crop Coefficient (Kcb + Ke)/Evaporation Component/Soil evaporation reduction coefficient (Kr)/REWmax total readily evaporable water [mm]/Ritchie et al. (1989) ==
  Add : Sum  Inputs=+++
  Compare To Constant : simulink/Logic and Bit Operations/Compare To Constant  relop=>=  const=0.8  OutDataTypeStr=boolean
  Compare To Constant1 : simulink/Logic and Bit Operations/Compare To Constant  relop=>=  const=0.5  OutDataTypeStr=boolean
  Compare To Constant2 : simulink/Logic and Bit Operations/Compare To Constant  relop=<  const=0.5  OutDataTypeStr=boolean
  Compare To Constant3 : simulink/Logic and Bit Operations/Compare To Constant  relop=<  const=0.8  OutDataTypeStr=boolean
  Constant : Constant  Value=20
  Constant1 : Constant  Value=11
  Constant2 : Constant  Value=8
  Gain : Gain  Gain=0.15
  Gain1 : Gain  Gain=0.06
  Gain2 : Gain  Gain=0.08
  Product : Product
  Product1 : Product
  Product2 : Product  Inputs=3
  Subtract : Sum  Inputs=+-
  Subtract1 : Sum  Inputs=+-
  Subtract2 : Sum  Inputs=+-
  Out1 : Outport
  wires:
  Compare To Constant3/1 -> Product2/3
  [PSand] -> Gain/1, Compare To Constant/1
  Subtract2/1 -> Product2/1
  Product/1 -> Add/1
  Product2/1 -> Add/3
  Gain/1 -> Subtract/2
  Compare To Constant/1 -> Product/2
  Subtract/1 -> Product/1
  Compare To Constant1/1 -> Product1/2
  Constant1/1 -> Subtract1/1
  Subtract1/1 -> Product1/1
  Gain2/1 -> Subtract2/2
  [PClay] -> Compare To Constant1/1, Gain1/1
  Constant2/1 -> Subtract2/1
  [PClay] -> Compare To Constant2/1, Gain2/1
  [PSand] -> Compare To Constant3/1
  Constant/1 -> Subtract/1
  Compare To Constant2/1 -> Product2/2
  Add/1 -> Out1/1
  Product1/1 -> Add/2
  Gain1/1 -> Subtract1/2

== system cop/COP/Soil Model/Soil Data Calculation/Estimated Soil Heat Capacity (UC Davis)/Bulk Density (Saxton and Rawls Function) [g//cm^3)/Normal Density (g//cm^3)/Saturated Moisture θS ==
  Constant : Constant  Value=0.097
  Constant1 : Constant  Value=0.043
  Product : Product
  Subtract : Sum  Inputs=++-+
  θ(S-33) : Subsystem
  Out1 : Outport
  wires:
  Subtract/1 -> Out1/1
  [qFC] -> Subtract/1
  Product/1 -> Subtract/3
  Constant/1 -> Product/1
  [PSand] -> Product/2
  Constant1/1 -> Subtract/4
  θ(S-33)/1(Out1) -> Subtract/2

== system cop/COP/Soil Model/Soil Data Calculation/Estimated Soil Heat Capacity (UC Davis)/Bulk Density (Saxton and Rawls Function) [g//cm^3)/Normal Density (g//cm^3)/Saturated Moisture θS/θ(S-33) ==
  Constant : Constant  Value=0.636
  Constant1 : Constant  Value=0.107
  Product : Product
  Subtract : Sum  Inputs=++-
  θ(S-33)t : Subsystem
  Out1 : Outport
  wires:
  θ(S-33)t/1(Out1) -> Product/1, Subtract/1
  Product/1 -> Subtract/2
  Constant/1 -> Product/2
  Constant1/1 -> Subtract/3
  Subtract/1 -> Out1/1

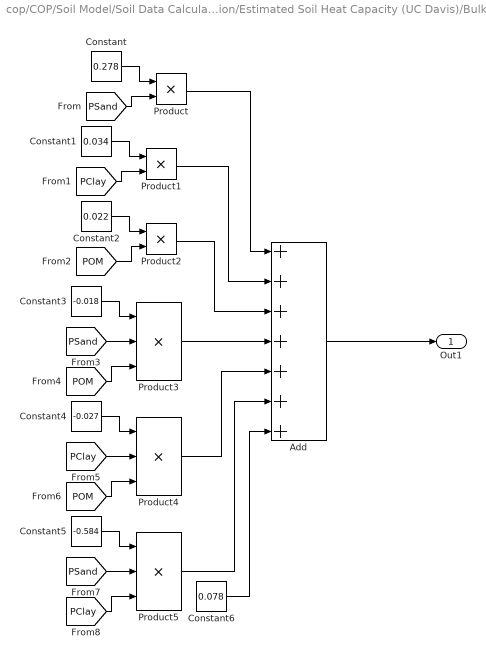
== system cop/COP/Soil Model/Soil Data Calculation/Estimated Soil Heat Capacity (UC Davis)/Bulk Density (Saxton and Rawls Function) [g//cm^3)/Normal Density (g//cm^3)/Saturated Moisture θS/θ(S-33)/θ(S-33)t ==
  Add : Sum  Inputs=+++++++
  Constant : Constant  Value=0.278
  Constant1 : Constant  Value=0.034
  Constant2 : Constant  Value=0.022
  Constant3 : Constant  Value=-0.018
  Constant4 : Constant  Value=-0.027
  Constant5 : Constant  Value=-0.584
  Constant6 : Constant  Value=0.078
  Product : Product
  Product1 : Product
  Product2 : Product
  Product3 : Product  Inputs=3
  Product4 : Product  Inputs=3
  Product5 : Product  Inputs=3
  Out1 : Outport
  wires:
  Add/1 -> Out1/1
  Constant2/1 -> Product2/1
  [POM] -> Product2/2
  Product1/1 -> Add/2
  Product2/1 -> Add/3
  [PClay] -> Product4/2
  Constant3/1 -> Product3/1
  [POM] -> Product3/3
  [PClay] -> Product1/2
  Constant6/1 -> Add/7
  Product5/1 -> Add/6
  [PClay] -> Product5/3
  Product/1 -> Add/1
  Constant5/1 -> Product5/1
  Constant1/1 -> Product1/1
  Constant/1 -> Product/1
  [POM] -> Product4/3
  Product3/1 -> Add/4
  [PSand] -> Product5/2
  [PSand] -> Product3/2
  Constant4/1 -> Product4/1
  [PSand] -> Product/2
  Product4/1 -> Add/5

== matlab function cop/COP/Plant Model/General Plant Database/MATLAB Function1 ==
  data: PDd input; cd output; PDm input; PDy input; DafterPD input; d output; m output; y output
function [cd,d,m,y] = curDate(PDd,PDm,PDy,DafterPD)
    x = datetime(PDy,PDm,PDd);
    x = x + floor(DafterPD);
    xv = datevec(x);
    y = xv(1);
    m = xv(2);
    d = xv(3);
    xm = datetime(y,1,1);
    a = minus(x,xm);
    cd = days(a);
end

== matlab function cop/COP/Plant Model/General Plant Database/MATLAB Function ==
  data: year input; D output
function D = DinYear(year)
    if mod(year, 4) == 0
        D = 366;
        if mod(year, 100) == 0
            D = 365;
            if mod(year,400)==0
                D = 366;
            end
        end
    else
        D = 365;
    end
end

== matlab function cop/COP/Plant Model/Plant Data Calculation/MATLAB Function ==
  data: d input; stage output; Lini input; Ldev input; Lmid input; Llate input
function stage = curPS(d,Lini,Ldev,Lmid,Llate)
    stage = 0;
    d = d - Lini;
    if d <= 0
        return
    end
    stage = 1;
    d = d - Ldev;
    if d <= 0
        return
    end
    stage = 2;
    d = d - Lmid;
    if d <= 0
        return
    end
    stage = 3;
    d = d - Lmid;
    if d <= 0 
        return
    end
    stage = 4;
end

== matlab function cop/COP/Soil Model/General Soil Database/MATLAB Function3 ==
  data: sand input; clay input; SC output; sand output; clay output; CMF output
function [SC,sand, clay, CMF] = soil_classification(sand, clay)

 if (sand + clay > 1) || sand<0 || clay<0
    error('data inconsisent: soil compositions need to sum to 1')
 end
%--------------------------------------------------------------------------
%--------------------------------------------------------------------------
%--------------------------------------------------------------------------
silt = 1 - sand - clay;
if (silt+1.5*clay)<.15
     SC ="SAND";
     CMF = 1;
 elseif ((silt+1.5*clay)>=.15)&&((silt+2*clay)<.3)
     SC ="LOAMY SAND";
     CMF = 1;
 elseif (clay>=0.07) && (clay<=0.2) && (sand>0.52) && ((silt+2*clay)>=0.3) 
     SC ="SANDY LOAM";
     CMF = 1;
 elseif (clay<0.07) && (silt < 0.5) && ((silt+2*clay)>=0.3)
     SC ="SANDY LOAM";
     CMF = 1;
 elseif (clay>=0.07) && (clay<=0.27) && (silt>=0.28) && (silt<0.5) && (sand<=0.52)
     SC ="LOAM";
     CMF = 2;
 elseif ((silt>=0.5) && clay>=0.12 && clay<0.27) || (silt>=0.5 && silt<0.8 && clay<0.12)
     SC ="SILT LOAM";
     CMF = 2;
 elseif silt>=0.8 && clay<0.12
     SC ="SILT";
     CMF = 2;
 elseif clay>=0.2 && clay<0.35 && silt<0.28 && sand>0.45
     SC ="SANDY CLAY LOAM";
     CMF = 2;
 elseif clay>=0.27 && clay <0.4 && sand>0.2 && sand<=0.45
     SC ="CLAY LOAM";
     CMF = 3;
 elseif clay>=0.27 && clay<0.4 && sand<=0.2
     SC ="SILTY CLAY LOAM";
     CMF = 3;
 elseif clay>=0.35 && sand>=0.45
     SC ="SANDY CLAY";
     CMF = 3;
 elseif clay>=0.4 && silt>=0.4
     SC ="SILTY CLAY";
     CMF = 3;
 elseif clay>= 0.4 && sand<=0.45 && silt<0.4
     SC ="CLAY";
     CMF = 3;
 else
     error('no soil class found')
end
end %of function
